simulink model "CIGRE_Islanded_1SM_2GFM_1GFL"  (R2020b)
settings: Solver=FixedStepAuto  StartTime=0.0  StopTime=simlt.T_stop  RelTol=1e-3
undefined symbols (not defined in the file): simlt
libraries: G2ELib_V1 x55, powerlib x19, powerlib_meascontrol x13, eePowerMeasurement x13
(part 2 of 2)

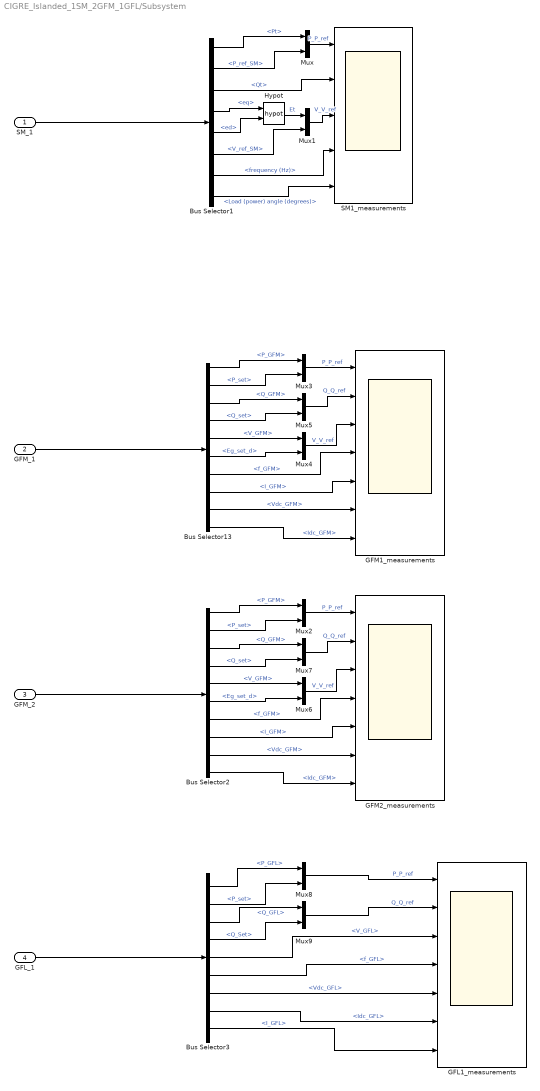
== system CIGRE_Islanded_1SM_2GFM_1GFL/Subsystem ==
  SM_1 : Inport
  GFM_1 : Inport  Port=2
  GFM_2 : Inport  Port=3
  GFL_1 : Inport  Port=4
  Bus Selector1 : BusSelector  OutputSignals=Terminal Powers (pu).Pt,References (P;V).P_ref_SM,Terminal Powers (pu).Qt,Terminal voltage dq-comp and field voltage (pu).eq,Terminal voltage dq-comp and field voltage (pu).ed,References (P;V).V_ref_SM,frequency (Hz),Load (power) angle (degrees)
  Bus Selector13 : BusSelector  OutputSignals=P_GFM,Setpoints.P_set,Q_GFM,Setpoints.Q_set,V_GFM,Setpoints.Eg_set_d,f_GFM,I_GFM,Vdc_GFM,Idc_GFM
  Bus Selector2 : BusSelector  OutputSignals=P_GFM,Setpoints.P_set,Q_GFM,Setpoints.Q_set,V_GFM,Setpoints.Eg_set_d,f_GFM,I_GFM,Vdc_GFM,Idc_GFM
  Bus Selector3 : BusSelector  OutputSignals=P_GFL,Setpoints.P_set,Q_GFL,Setpoints.Q_Set,V_GFL,f_GFL,Vdc_GFL,Idc_GFL,I_GFL
  GFL1_measurements : Scope  NumInputPorts=7
  GFM1_measurements : Scope  NumInputPorts=7
  GFM2_measurements : Scope  NumInputPorts=7
  Hypot : Math  Operator=hypot  SaturateOnIntegerOverflow=on
  Mux{,1..9} (10 alike) : Mux  Inputs=2
  SM1_measurements : Scope  NumInputPorts=5
  wires:
  SM_1/1 -> Bus Selector1/1
  Mux1/1 -> SM1_measurements/3  "V_V_ref"
  Hypot/1 -> Mux1/1  "Et"
  Bus Selector1/3 -> SM1_measurements/2  "<Qt>"
  Bus Selector1/4 -> Hypot/1  "<eq>"
  Bus Selector1/6 -> Mux1/2  "<V_ref_SM>"
  Mux/1 -> SM1_measurements/1  "P_P_ref"
  Bus Selector1/7 -> SM1_measurements/4  "<frequency (Hz)>"
  Bus Selector1/8 -> SM1_measurements/5  "<Load (power) angle (degrees)>"
  Bus Selector1/1 -> Mux/1  "<Pt>"
  Bus Selector1/2 -> Mux/2  "<P_ref_SM>"
  Bus Selector1/5 -> Hypot/2  "<ed>"
  Mux4/1 -> GFM1_measurements/3  "V_V_ref"
  Bus Selector13/5 -> Mux4/1  "<V_GFM>"
  Bus Selector13/4 -> Mux5/2  "<Q_set>"
  Bus Selector13/7 -> GFM1_measurements/4  "<f_GFM>"
  Mux3/1 -> GFM1_measurements/1  "P_P_ref"
  Bus Selector13/1 -> Mux3/1  "<P_GFM>"
  GFM_1/1 -> Bus Selector13/1
  Mux5/1 -> GFM1_measurements/2  "Q_Q_ref"
  Bus Selector13/2 -> Mux3/2  "<P_set>"
  Bus Selector13/10 -> GFM1_measurements/7  "<Idc_GFM>"
  Bus Selector13/8 -> GFM1_measurements/5  "<I_GFM>"
  Bus Selector13/3 -> Mux5/1  "<Q_GFM>"
  Bus Selector13/9 -> GFM1_measurements/6  "<Vdc_GFM>"
  Bus Selector13/6 -> Mux4/2  "<Eg_set_d>"
  Bus Selector2/6 -> Mux6/2  "<Eg_set_d>"
  Bus Selector2/9 -> GFM2_measurements/6  "<Vdc_GFM>"
  Bus Selector2/3 -> Mux7/1  "<Q_GFM>"
  Bus Selector2/8 -> GFM2_measurements/5  "<I_GFM>"
  Bus Selector2/10 -> GFM2_measurements/7  "<Idc_GFM>"
  Bus Selector2/2 -> Mux2/2  "<P_set>"
  Mux7/1 -> GFM2_measurements/2  "Q_Q_ref"
  GFM_2/1 -> Bus Selector2/1
  Bus Selector2/1 -> Mux2/1  "<P_GFM>"
  Mux2/1 -> GFM2_measurements/1  "P_P_ref"
  Bus Selector2/7 -> GFM2_measurements/4  "<f_GFM>"
  Bus Selector2/4 -> Mux7/2  "<Q_set>"
  Bus Selector2/5 -> Mux6/1  "<V_GFM>"
  Mux6/1 -> GFM2_measurements/3  "V_V_ref"
  Bus Selector3/3 -> Mux9/1  "<Q_GFL>"
  Mux8/1 -> GFL1_measurements/1  "P_P_ref"
  Bus Selector3/2 -> Mux8/2  "<P_set>"
  Bus Selector3/9 -> GFL1_measurements/7  "<I_GFL>"
  Bus Selector3/7 -> GFL1_measurements/5  "<Vdc_GFL>"
  Bus Selector3/5 -> GFL1_measurements/3  "<V_GFL>"
  Bus Selector3/8 -> GFL1_measurements/6  "<Idc_GFL>"
  GFL_1/1 -> Bus Selector3/1
  Bus Selector3/4 -> Mux9/2  "<Q_Set>"
  Bus Selector3/1 -> Mux8/1  "<P_GFL>"
  Bus Selector3/6 -> GFL1_measurements/4  "<f_GFL>"
  Mux9/1 -> GFL1_measurements/2  "Q_Q_ref"
